simulink model "RobotX_JacobSimul"  (R2024a)
settings: Solver=VariableStepAuto  StartTime=0.0  StopTime=10.0  MaxStep=1e-5  RelTol=1e-3
libraries: RobotX_Lib x1, matrix_library x1
settings Model: PacingRate=0.010000  Creator=margaridaestrela  LastModifiedBy=margaridaestrela

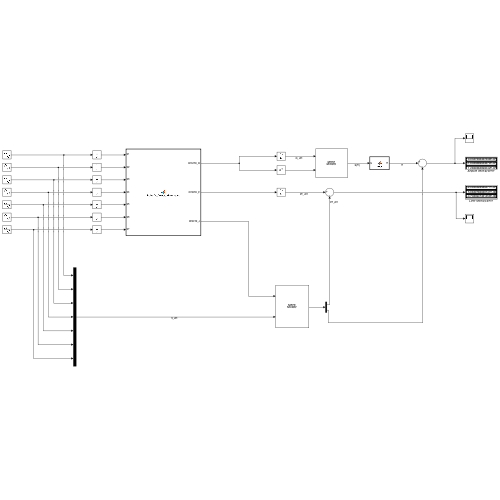
[thumbnail: Simulink's stored preview of the top-level diagram]
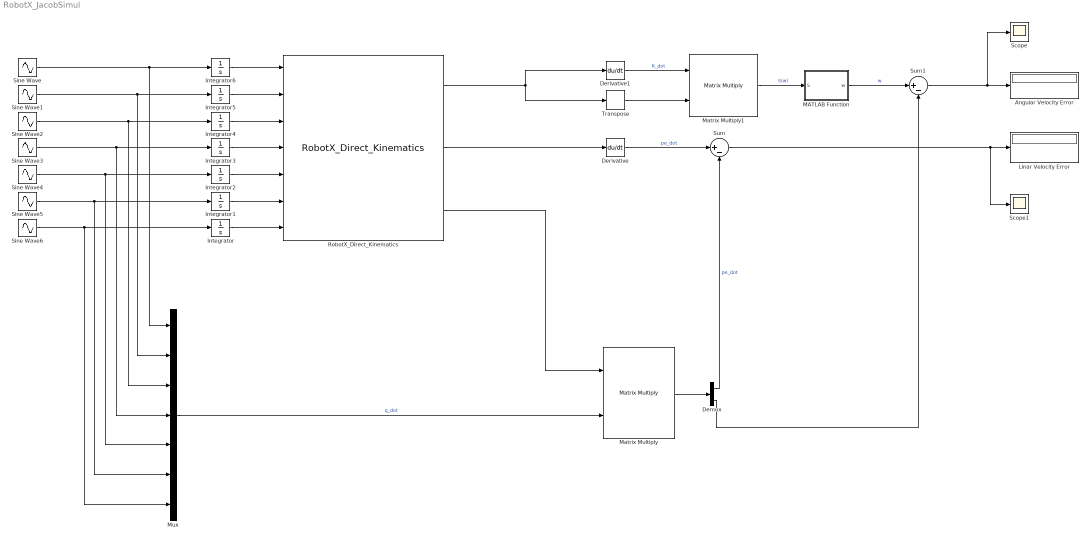
== system RobotX_JacobSimul ==
  Angular Velocity Error : Display
      settings: Format=decimal (Stored Integer)  Decimation=2
  Demux : Demux  Outputs=2
  Derivative : Derivative
  Derivative1 : Derivative
  Integrator{,1..6} (7 alike) : Integrator
  Linar Velocity Error : Display
      settings: Format=decimal (Stored Integer)  Decimation=2
  MATLAB Function : MATLAB Function  TreatAsAtomicUnit=on
  Matrix Multiply : Product  Multiplication=Matrix(*)
  Matrix Multiply1 : Product  Multiplication=Matrix(*)
  Mux : Mux  Inputs=7
  RobotX_Direct_Kinematics : RobotX_Lib/RobotX_Direct_Kinematics  SystemSampleTime=-1  VariantActivationTime=update diagram  AllowFlexibleInterface=on  Latency=0  AutoFrameSizeCalculation=off
  Scope : Scope
  Scope1 : Scope
  Sine Wave{,1..6} (7 alike) : Sin  SampleTime=0
  Sum : Sum  Inputs=|+-
  Sum1 : Sum  Inputs=|+-
  Transpose : matrix_library/Transpose
  wires:
  Integrator2/1 -> RobotX_Direct_Kinematics/5
  Integrator1/1 -> RobotX_Direct_Kinematics/6
  Integrator3/1 -> RobotX_Direct_Kinematics/4
  Integrator4/1 -> RobotX_Direct_Kinematics/3
  Integrator6/1 -> RobotX_Direct_Kinematics/1
  Integrator5/1 -> RobotX_Direct_Kinematics/2
  RobotX_Direct_Kinematics/3 -> Matrix Multiply/1
  Mux/1 -> Matrix Multiply/2  "q_dot"
  RobotX_Direct_Kinematics/2 -> Derivative/1
  Derivative/1 -> Sum/1  "pe_dot"
  Sum/1 -> Scope1/1, Linar Velocity Error/1
  Demux/1 -> Sum/2  "pe_dot"
  RobotX_Direct_Kinematics/1 -> Transpose/1, Derivative1/1
  Derivative1/1 -> Matrix Multiply1/1  "R_dot"
  Transpose/1 -> Matrix Multiply1/2
  Matrix Multiply1/1 -> MATLAB Function/1(S)  "S(w)"
  MATLAB Function/1(w) -> Sum1/1  "w"
  Sum1/1 -> Scope/1, Angular Velocity Error/1
  Sine Wave1/1 -> Integrator5/1, Mux/2
  Sine Wave2/1 -> Integrator4/1, Mux/3
  Sine Wave3/1 -> Integrator3/1, Mux/4
  Sine Wave4/1 -> Integrator2/1, Mux/5
  Sine Wave5/1 -> Integrator1/1, Mux/6
  Sine Wave6/1 -> Integrator/1, Mux/7
  Sine Wave/1 -> Mux/1, Integrator6/1
  Integrator/1 -> RobotX_Direct_Kinematics/7
  Demux/2 -> Sum1/2
  Matrix Multiply/1 -> Demux/1

== matlab function RobotX_JacobSimul/MATLAB Function ==
  data: S input; w output
function w = vect(S)

w = [S(3,2); S(1,3); S(2,1)];
